simulink model "qss_example_conv"  (Simulink 8.3)
settings: Solver=VariableStepDiscrete  StartTime=0.0  StopTime=1220  RelTol=1e-3
libraries: qss_tb_library_aalto x5
settings Model: Creator=Antti  LastModifiedBy=alajunen
settings DataIOCC: LimitDataPoints=off  SaveOutput=off  SaveTime=off
settings OptimizationCC: ExpressionDepthLimit=2147483647  InitFltsAndDblsToZero=on
settings DebuggingCC: SaveWithParameterizedLinksMsg=none  SignalResolutionControl=TryResolveAllWithWarning  MultiTaskDSMMsg=warning  MultiTaskCondExecSysMsg=none  FcnCallInpInsideContextMsg=UseLocalSettings
settings RTWCC: IncludeERTFirstTime=on
settings GRTTargetCC: TargetFcnLib=ansi_tfl_tmw.mat

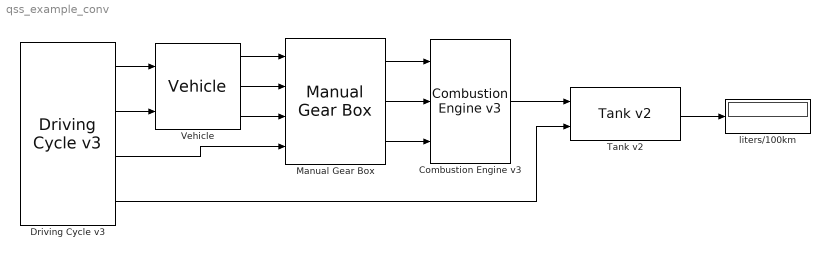
== system qss_example_conv ==
  Combustion Engine v3 : qss_tb_library_aalto/Energy Converter/Combustion Engine v3  Tag=combustion engine  engine_type=Otto  V_d=1.9  theta_CE=0.1  w_CE_idle=105  P_CE_idle=0  P_aux=300  ENABLE_FUEL_CUTOFF=on  T_CE_cutoff=2  P_CE_cutoff=0
  Driving Cycle v3 : qss_tb_library_aalto/Driving Cycle/Driving Cycle v3  Tag=cycle  cyclenr=Europe: NEDC  stepsize=1  autostop=on
  Manual Gear Box : qss_tb_library_aalto/Gear System/Manual Gear Box  Tag=transmission  i_1=15.174  i_2=8.338  i_3=5.378  i_4=3.937  i_5=2.748  i_diff=1  e_GT=0.98  P_GT0=300  w_wheel_min=1
  Tank v2 : qss_tb_library_aalto/Energy Source/Tank v2  Tag=tank  flag_cold_start=off
  Vehicle : qss_tb_library_aalto/Vehicle/Vehicle  Tag=vehicle  m_f=1200  mt2m_f=5  A_f=2.0  d_wheel=0.6  cw=0.33  mu=0.01
  liters/100km : Display
  wires:
  Driving Cycle v3/1 -> Vehicle/1
  Vehicle/1 -> Manual Gear Box/1
  Vehicle/2 -> Manual Gear Box/2
  Vehicle/3 -> Manual Gear Box/3
  Driving Cycle v3/2 -> Vehicle/2
  Manual Gear Box/1 -> Combustion Engine v3/1
  Manual Gear Box/2 -> Combustion Engine v3/2
  Manual Gear Box/3 -> Combustion Engine v3/3
  Driving Cycle v3/3 -> Manual Gear Box/4
  Driving Cycle v3/4 -> Tank v2/2
  Combustion Engine v3/1 -> Tank v2/1
  Tank v2/1 -> liters/100km/1
